simulink model "echo_inf_model"  (R2022b)
settings: Solver=VariableStepAuto  StartTime=0.0  StopTime=10.0  RelTol=1e-3
settings Model: Creator=berka  LastModifiedBy=berka

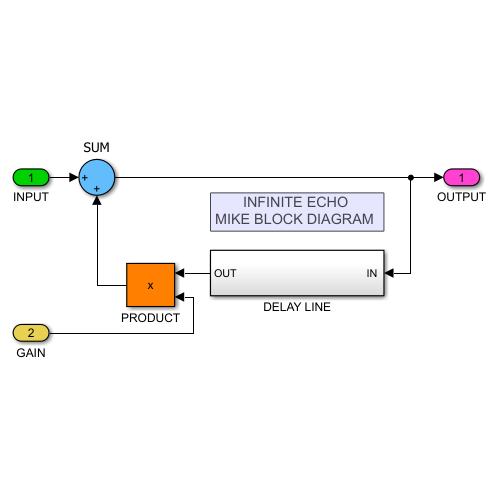
[thumbnail: Simulink's stored preview of the top-level diagram]
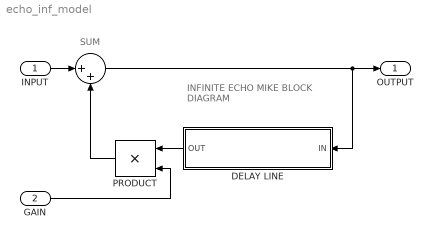
== system echo_inf_model ==
  note: INFINITE ECHO
      | MIKE BLOCK DIAGRAM
  note: SUM
  INPUT : Inport
  GAIN : Inport  Port=2
  " " : Sum  Inputs=|++
  DELAY LINE : Subsystem
  PRODUCT : Product
  OUTPUT : Outport
  wires:
  INPUT/1 -> " "/1
  " "/1 -> DELAY LINE/1("IN "), OUTPUT/1
  PRODUCT/1 -> " "/2
  DELAY LINE/1(OUT) -> PRODUCT/1
  GAIN/1 -> PRODUCT/2

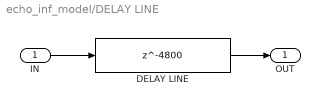
== system echo_inf_model/DELAY LINE ==
  "IN " : Inport
  DELAY LINE : Delay  DelayLength=4800  InitialCondition=0
  OUT : Outport
  wires:
  "IN "/1 -> DELAY LINE/1
  DELAY LINE/1 -> OUT/1
